simulink model "orbit_propogator_num"  (R2023b)
settings: Solver=ode4  StartTime=0  StopTime=Tfinal  FixedStep=50  RelTol=1e-3
settings Model: Creator=annahylbert  LastModifiedBy=kristopherriordan

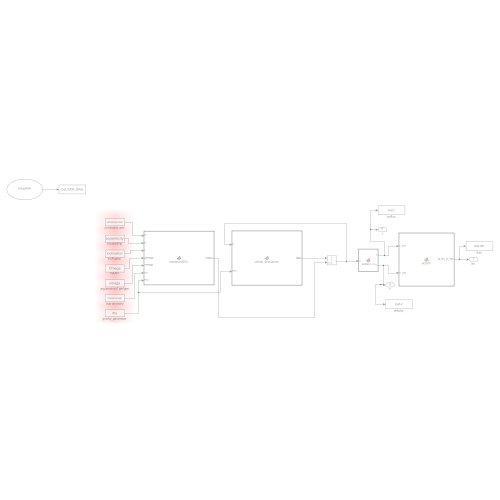
[thumbnail: Simulink's stored preview of the top-level diagram]
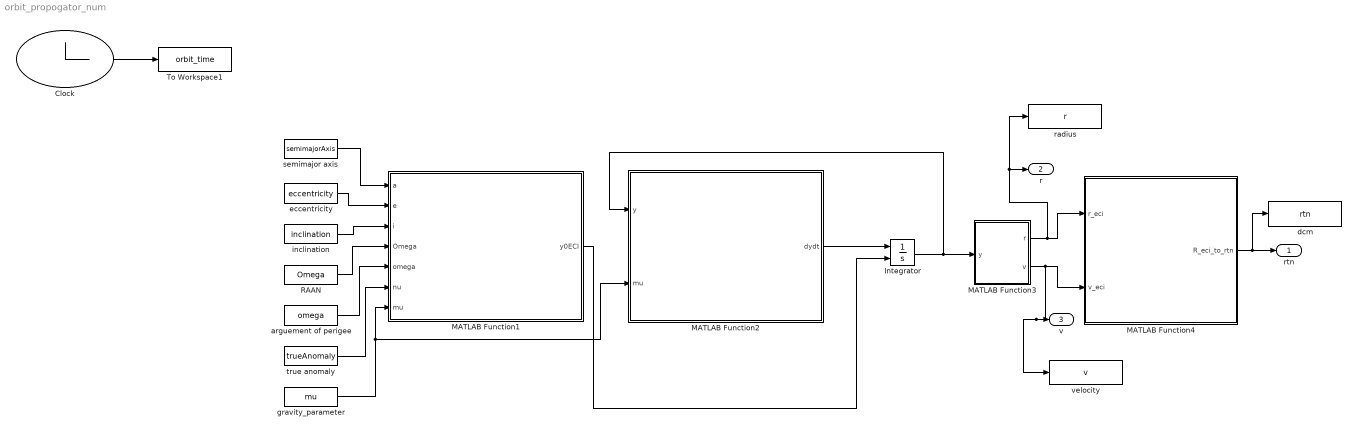
== system orbit_propogator_num ==
  Clock : Clock
      settings: Decimation=99999999
  Integrator : Integrator  InitialConditionSource=external
  MATLAB Function1 : MATLAB Function  TreatAsAtomicUnit=on
  MATLAB Function2 : MATLAB Function  TreatAsAtomicUnit=on
  MATLAB Function3 : MATLAB Function  TreatAsAtomicUnit=on
  MATLAB Function4 : MATLAB Function  TreatAsAtomicUnit=on
  RAAN : FromWorkspace  VariableName=Omega
  To Workspace1 : ToWorkspace  VariableName=orbit_time  SaveFormat=Timeseries  SampleTime=-1
  arguement of perigee : FromWorkspace  VariableName=omega
  dcm : ToWorkspace  VariableName=rtn  SaveFormat=Timeseries  SampleTime=-1
  eccentricity : FromWorkspace  VariableName=eccentricity
  gravity_parameter : FromWorkspace  VariableName=mu
  inclination : FromWorkspace  VariableName=inclination
  radius : ToWorkspace  VariableName=r  SaveFormat=Timeseries  SampleTime=-1
  semimajor axis : FromWorkspace  VariableName=semimajorAxis  OutDataTypeStr=double
  true anomaly : FromWorkspace  VariableName=trueAnomaly
  velocity : ToWorkspace  VariableName=v  SaveFormat=Timeseries  SampleTime=-1
  rtn : Outport
  r : Outport  Port=2
  v : Outport  Port=3
  wires:
  eccentricity/1 -> MATLAB Function1/2(e)
  semimajor axis/1 -> MATLAB Function1/1(a)
  inclination/1 -> MATLAB Function1/3(i)
  RAAN/1 -> MATLAB Function1/4(Omega)
  arguement of perigee/1 -> MATLAB Function1/5(omega)
  Clock/1 -> To Workspace1/1
  true anomaly/1 -> MATLAB Function1/6(nu)
  gravity_parameter/1 -> MATLAB Function2/2(mu), MATLAB Function1/7(mu)
  MATLAB Function2/1(dydt) -> Integrator/1
  MATLAB Function1/1(y0ECI) -> Integrator/2
  Integrator/1 -> MATLAB Function3/1(y), MATLAB Function2/1(y)
  MATLAB Function3/1(r) -> radius/1, r/1, MATLAB Function4/1(r_eci)
  MATLAB Function3/2(v) -> velocity/1, v/1, MATLAB Function4/2(v_eci)
  MATLAB Function4/1(R_eci_to_rtn) -> dcm/1, rtn/1

== matlab function orbit_propogator_num/MATLAB Function1 ==
  data: a input; y0ECI output; e input; i input; Omega input; omega input; nu input; mu input
function y0ECI = keplerian2ECI(a, e, i, Omega, omega, nu, mu)

    % Calculate position and velocity in the perifocal coordinate system
    E = acos((e + cos(nu))/(1+(e*cos(nu))));
    n = sqrt(mu/a^3);
    r_perifocal = [a*(cos(E) - e); a*sin(E)*sqrt(1-e^2); 0];
    v_perifocal = a*n/(1-e*cos(E)) * [-sin(E); cos(E)*sqrt(1-e^2); 0];

    % Rotation matrices
    R3_Omega = [cos(-Omega) sin(-Omega) 0;
                -sin(-Omega) cos(-Omega) 0;
                0 0 1];
    R1_i = [1 0 0;
            0 cos(-i) sin(-i);
            0 -sin(-i) cos(-i)];
    R3_omega = [cos(-omega) sin(-omega) 0;
                -sin(-omega) cos(-omega) 0;
                0 0 1];

    % Transformation to ECI
    Q_perifocal2ECI = R3_Omega * R1_i * R3_omega;
    r0 = Q_perifocal2ECI * r_perifocal;
    v0 = Q_perifocal2ECI * v_perifocal;

    y0ECI = [r0; v0];
end

== matlab function orbit_propogator_num/MATLAB Function2 ==
  data: dydt output; y input; mu input
function dydt = orbital_derivatives(y, mu)
    % Define the equations of motion for orbital derivatives
    r = y(1:3);
    v = y(4:6);
    r_mag = norm(r);
    dvdt = -mu * r / r_mag^3;
    drdt = v;
    dydt = [drdt; dvdt];
end

== matlab function orbit_propogator_num/MATLAB Function3 ==
  data: r output; y input; v output
function [r,v] = extract_rv(y)
    % Define the equations of motion for orbital derivatives
    r = y(1:3);
    v = y(4:6);
end

== matlab function orbit_propogator_num/MATLAB Function4 ==
  data: R_eci_to_rtn output; r_eci input; v_eci input
function R_eci_to_rtn = eci2rtn(r_eci, v_eci)
    
    % Compute radial, transverse, and normal vectors in ECI frame
    r_radial_eci = r_eci;
    r_normal_eci = cross(r_radial_eci, v_eci);
    r_transverse_eci = -cross(r_radial_eci, r_normal_eci);
    
    % Normalize radial, transverse, and normal vectors to obtain unit vectors
    r_radial_eci_unit = r_radial_eci / norm(r_radial_eci);
    r_transverse_eci_unit = r_transverse_eci / norm(r_transverse_eci);
    r_normal_eci_unit = r_normal_eci / norm(r_normal_eci);
    
    % Construct rotation matrix from ECI to RTN
    R_eci_to_rtn = [r_radial_eci_unit.'; r_transverse_eci_unit.'; r_normal_eci_unit.'];

end
